simulink model "nn_fuel_control_4_20"  (R2021a)
settings: Solver=ode15s  StartTime=0.0  StopTime=T  MaxStep=.01  RelTol=1e-3
undefined symbols (not defined in the file): AF_sensor_tol, fault_time, fuel_inj_tol, kappa_tol, MAF_sensor_tol, pump_tol, tau_ww_tol
libraries: neural x86
(part 2 of 4)

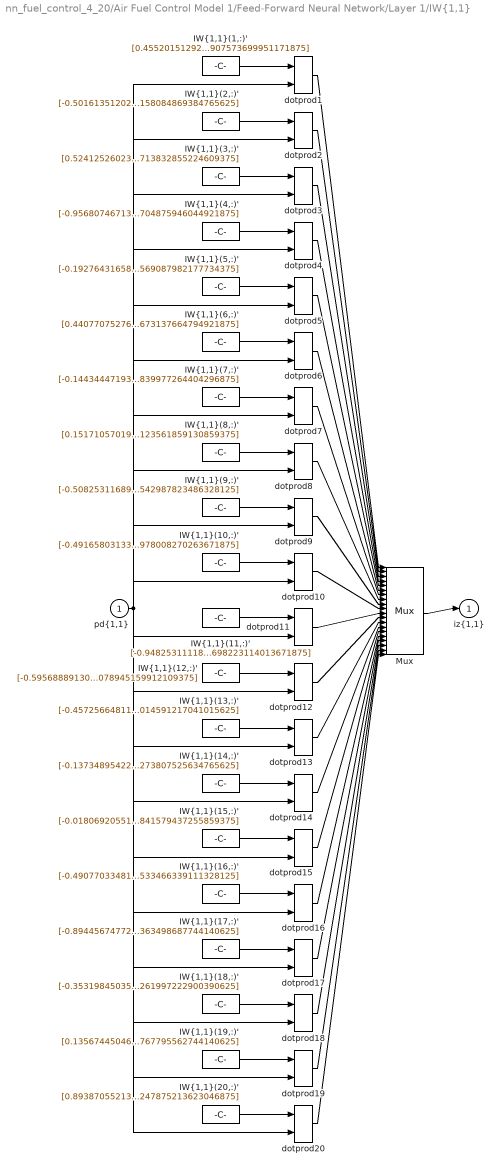
== system nn_fuel_control_4_20/Air Fuel Control Model 1/Feed-Forward Neural Network/Layer 1/IW{1,1} ==
  "pd{1,1}" : Inport  PortDimensions=4
      mask Display: e = 0.06;c1 = [120 230 180]/255;c2 = ([120 230 180]+0)/(256+128);c3 = ([120 230 180]+128)/(256+128);patch([0 1 1 0],[0 0 1 1],c1);patch([0 1 1 1-e 1-e 0+e],[0 0 1 1-e 0+e 0+e],c2);patch([0 0 1 1-e 0+e 0+e],[0 1 1 1-e 1-e 0+e],c3);plot([0 1 1 0 0],[0 0 1 1 0]);
  "IW{1,1}(1,:)'" : Constant  Value=[0.455201512923426532264414845485589466989040374755859375;0.6210675018319438134284382613259367644786834716796875;0.08959089907253227347272428460200899280607700347900390625;1.050437900131484081356347815017215907573699951171875]
      mask Display: e = 0.06;c1 = [120 150 230]/255;c2 = ([120 150 230]+0)/383;c3 = ([120 150 230]+128)/383;patch([0 1 1 0],[0 0 1 1],c1);patch([0 1 1 1-e 1-e 0+e],[0 0 1 1-e 0+e 0+e],c2);patch([0 0 1 1-e 0+e 0+e],[0 1 1 1-e 1-e 0+e],c3);plot([0 1 1 0 0],[0 0 1 1 0]);disp('Weights');
  "IW{1,1}(10,:)'" : Constant  Value=[-0.4916580313329574902780905176769010722637176513671875;0.71234771766081284027904985123313963413238525390625;-0.7859957167075719564053315480123274028301239013671875;0.114661304117702922411581312189809978008270263671875]
      mask Display: e = 0.06;c1 = [120 150 230]/255;c2 = ([120 150 230]+0)/383;c3 = ([120 150 230]+128)/383;patch([0 1 1 0],[0 0 1 1],c1);patch([0 1 1 1-e 1-e 0+e],[0 0 1 1-e 0+e 0+e],c2);patch([0 0 1 1-e 0+e 0+e],[0 1 1 1-e 1-e 0+e],c3);plot([0 1 1 0 0],[0 0 1 1 0]);disp('Weights');
  "IW{1,1}(11,:)'" : Constant  Value=[-0.9482531111801184575682555077946744859218597412109375;0.48788166885906480985113375936634838581085205078125;-0.87517942770330936497202856116928160190582275390625;0.5022120925968749372003685493837110698223114013671875]
      mask Display: e = 0.06;c1 = [120 150 230]/255;c2 = ([120 150 230]+0)/383;c3 = ([120 150 230]+128)/383;patch([0 1 1 0],[0 0 1 1],c1);patch([0 1 1 1-e 1-e 0+e],[0 0 1 1-e 0+e 0+e],c2);patch([0 0 1 1-e 0+e 0+e],[0 1 1 1-e 1-e 0+e],c3);plot([0 1 1 0 0],[0 0 1 1 0]);disp('Weights');
  "IW{1,1}(12,:)'" : Constant  Value=[-0.59568889130134561327167830313555896282196044921875;0.3387998983611222314493716112338006496429443359375;0.009359495090498715086368974880315363407135009765625;-0.4969588631373615950082012204802595078945159912109375]
      mask Display: e = 0.06;c1 = [120 150 230]/255;c2 = ([120 150 230]+0)/383;c3 = ([120 150 230]+128)/383;patch([0 1 1 0],[0 0 1 1],c1);patch([0 1 1 1-e 1-e 0+e],[0 0 1 1-e 0+e 0+e],c2);patch([0 0 1 1-e 0+e 0+e],[0 1 1 1-e 1-e 0+e],c3);plot([0 1 1 0 0],[0 0 1 1 0]);disp('Weights');
  "IW{1,1}(13,:)'" : Constant  Value=[-0.457256648119046371636642334124189801514148712158203125;0.357249947753426611019023084736545570194721221923828125;-0.57752587680887235155324788138386793434619903564453125;0.8892340081964162923355843304307200014591217041015625]
      mask Display: e = 0.06;c1 = [120 150 230]/255;c2 = ([120 150 230]+0)/383;c3 = ([120 150 230]+128)/383;patch([0 1 1 0],[0 0 1 1],c1);patch([0 1 1 1-e 1-e 0+e],[0 0 1 1-e 0+e 0+e],c2);patch([0 0 1 1-e 0+e 0+e],[0 1 1 1-e 1-e 0+e],c3);plot([0 1 1 0 0],[0 0 1 1 0]);disp('Weights');
  "IW{1,1}(14,:)'" : Constant  Value=[-0.1373489542293671039629998631426133215427398681640625;-0.5775747421829160455075680147274397313594818115234375;-0.738357415907519243347678639111109077930450439453125;-0.697311127666600416574738119379617273807525634765625]
      mask Display: e = 0.06;c1 = [120 150 230]/255;c2 = ([120 150 230]+0)/383;c3 = ([120 150 230]+128)/383;patch([0 1 1 0],[0 0 1 1],c1);patch([0 1 1 1-e 1-e 0+e],[0 0 1 1-e 0+e 0+e],c2);patch([0 0 1 1-e 0+e 0+e],[0 1 1 1-e 1-e 0+e],c3);plot([0 1 1 0 0],[0 0 1 1 0]);disp('Weights');
  "IW{1,1}(15,:)'" : Constant  Value=[-0.0180692055168433750311773877683663158677518367767333984375;0.21992142303115691515102980702067725360393524169921875;0.1282003875108993773412890959662036038935184478759765625;0.259471893671093523092707755495212040841579437255859375]
      mask Display: e = 0.06;c1 = [120 150 230]/255;c2 = ([120 150 230]+0)/383;c3 = ([120 150 230]+128)/383;patch([0 1 1 0],[0 0 1 1],c1);patch([0 1 1 1-e 1-e 0+e],[0 0 1 1-e 0+e 0+e],c2);patch([0 0 1 1-e 0+e 0+e],[0 1 1 1-e 1-e 0+e],c3);plot([0 1 1 0 0],[0 0 1 1 0]);disp('Weights');
  "IW{1,1}(16,:)'" : Constant  Value=[-0.4907703348185261660319156362675130367279052734375;-0.0863636826544158520135852086241357028484344482421875;-0.960556512884881197322783918934874236583709716796875;-0.0353694437489793234163926172186620533466339111328125]
      mask Display: e = 0.06;c1 = [120 150 230]/255;c2 = ([120 150 230]+0)/383;c3 = ([120 150 230]+128)/383;patch([0 1 1 0],[0 0 1 1],c1);patch([0 1 1 1-e 1-e 0+e],[0 0 1 1-e 0+e 0+e],c2);patch([0 0 1 1-e 0+e 0+e],[0 1 1 1-e 1-e 0+e],c3);plot([0 1 1 0 0],[0 0 1 1 0]);disp('Weights');
  "IW{1,1}(17,:)'" : Constant  Value=[-0.8944567477260270127459307332173921167850494384765625;-0.74001304047881399927888423917465843260288238525390625;-0.158439343135515942062596650430350564420223236083984375;0.5537273793157526657893185983994044363498687744140625]
      mask Display: e = 0.06;c1 = [120 150 230]/255;c2 = ([120 150 230]+0)/383;c3 = ([120 150 230]+128)/383;patch([0 1 1 0],[0 0 1 1],c1);patch([0 1 1 1-e 1-e 0+e],[0 0 1 1-e 0+e 0+e],c2);patch([0 0 1 1-e 0+e 0+e],[0 1 1 1-e 1-e 0+e],c3);plot([0 1 1 0 0],[0 0 1 1 0]);disp('Weights');
  "IW{1,1}(18,:)'" : Constant  Value=[-0.353198450357381066311290851444937288761138916015625;0.325674444826059339419543903204612433910369873046875;-0.9634401645374384148823310169973410665988922119140625;-0.0229134503222321317394971629255451261997222900390625]
      mask Display: e = 0.06;c1 = [120 150 230]/255;c2 = ([120 150 230]+0)/383;c3 = ([120 150 230]+128)/383;patch([0 1 1 0],[0 0 1 1],c1);patch([0 1 1 1-e 1-e 0+e],[0 0 1 1-e 0+e 0+e],c2);patch([0 0 1 1-e 0+e 0+e],[0 1 1 1-e 1-e 0+e],c3);plot([0 1 1 0 0],[0 0 1 1 0]);disp('Weights');
  "IW{1,1}(19,:)'" : Constant  Value=[0.135674450466279516991363607303355820477008819580078125;-0.549322912787994166450289412750862538814544677734375;-0.471953594740415038888414756002021022140979766845703125;0.1558695073946478049098374185632565058767795562744140625]
      mask Display: e = 0.06;c1 = [120 150 230]/255;c2 = ([120 150 230]+0)/383;c3 = ([120 150 230]+128)/383;patch([0 1 1 0],[0 0 1 1],c1);patch([0 1 1 1-e 1-e 0+e],[0 0 1 1-e 0+e 0+e],c2);patch([0 0 1 1-e 0+e 0+e],[0 1 1 1-e 1-e 0+e],c3);plot([0 1 1 0 0],[0 0 1 1 0]);disp('Weights');
  "IW{1,1}(2,:)'" : Constant  Value=[-0.50161351202444370844801824205205775797367095947265625;0.958190578215499133563071154640056192874908447265625;-0.056301596982187458728663642659739707596600055694580078125;0.040480469393256370003175703686792985536158084869384765625]
      mask Display: e = 0.06;c1 = [120 150 230]/255;c2 = ([120 150 230]+0)/383;c3 = ([120 150 230]+128)/383;patch([0 1 1 0],[0 0 1 1],c1);patch([0 1 1 1-e 1-e 0+e],[0 0 1 1-e 0+e 0+e],c2);patch([0 0 1 1-e 0+e 0+e],[0 1 1 1-e 1-e 0+e],c3);plot([0 1 1 0 0],[0 0 1 1 0]);disp('Weights');
  "IW{1,1}(20,:)'" : Constant  Value=[0.8938705521315066793164305636310018599033355712890625;0.96329793238814798161939734200132079422473907470703125;-0.295572392642879544499834310045116581022739410400390625;0.87909372842644284418156530591659247875213623046875]
      mask Display: e = 0.06;c1 = [120 150 230]/255;c2 = ([120 150 230]+0)/383;c3 = ([120 150 230]+128)/383;patch([0 1 1 0],[0 0 1 1],c1);patch([0 1 1 1-e 1-e 0+e],[0 0 1 1-e 0+e 0+e],c2);patch([0 0 1 1-e 0+e 0+e],[0 1 1 1-e 1-e 0+e],c3);plot([0 1 1 0 0],[0 0 1 1 0]);disp('Weights');
  "IW{1,1}(3,:)'" : Constant  Value=[0.5241252602301378349380911458865739405155181884765625;0.8167734373000536951536787455552257597446441650390625;-0.74201764338017017763604599167592823505401611328125;-0.832946956754459844063376294798217713832855224609375]
      mask Display: e = 0.06;c1 = [120 150 230]/255;c2 = ([120 150 230]+0)/383;c3 = ([120 150 230]+128)/383;patch([0 1 1 0],[0 0 1 1],c1);patch([0 1 1 1-e 1-e 0+e],[0 0 1 1-e 0+e 0+e],c2);patch([0 0 1 1-e 0+e 0+e],[0 1 1 1-e 1-e 0+e],c3);plot([0 1 1 0 0],[0 0 1 1 0]);disp('Weights');
  "IW{1,1}(4,:)'" : Constant  Value=[-0.956807467135799782909089117310941219329833984375;-0.0493903087290285258692534853253164328634738922119140625;-0.9415456718123842438927795228664763271808624267578125;-0.030347378954881314150338056379041518084704875946044921875]
      mask Display: e = 0.06;c1 = [120 150 230]/255;c2 = ([120 150 230]+0)/383;c3 = ([120 150 230]+128)/383;patch([0 1 1 0],[0 0 1 1],c1);patch([0 1 1 1-e 1-e 0+e],[0 0 1 1-e 0+e 0+e],c2);patch([0 0 1 1-e 0+e 0+e],[0 1 1 1-e 1-e 0+e],c3);plot([0 1 1 0 0],[0 0 1 1 0]);disp('Weights');
  "IW{1,1}(5,:)'" : Constant  Value=[-0.192764316586044592849447099069948308169841766357421875;-0.68996992127067391376016303183860145509243011474609375;0.354029156232344377475129704180289991199970245361328125;-0.08997556570563967903719770902171148918569087982177734375]
      mask Display: e = 0.06;c1 = [120 150 230]/255;c2 = ([120 150 230]+0)/383;c3 = ([120 150 230]+128)/383;patch([0 1 1 0],[0 0 1 1],c1);patch([0 1 1 1-e 1-e 0+e],[0 0 1 1-e 0+e 0+e],c2);patch([0 0 1 1-e 0+e 0+e],[0 1 1 1-e 1-e 0+e],c3);plot([0 1 1 0 0],[0 0 1 1 0]);disp('Weights');
  "IW{1,1}(6,:)'" : Constant  Value=[0.440770752766682705203749037536908872425556182861328125;0.1872641645973948387737806342556723393499851226806640625;0.46877269832112744563090700467000715434551239013671875;0.09773402402077450978890027499801362864673137664794921875]
      mask Display: e = 0.06;c1 = [120 150 230]/255;c2 = ([120 150 230]+0)/383;c3 = ([120 150 230]+128)/383;patch([0 1 1 0],[0 0 1 1],c1);patch([0 1 1 1-e 1-e 0+e],[0 0 1 1-e 0+e 0+e],c2);patch([0 0 1 1-e 0+e 0+e],[0 1 1 1-e 1-e 0+e],c3);plot([0 1 1 0 0],[0 0 1 1 0]);disp('Weights');
  "IW{1,1}(7,:)'" : Constant  Value=[-0.1443444719366482609235191603147541172802448272705078125;0.142050703362333441415188417522585950791835784912109375;-0.81241480909466534665597237108158878982067108154296875;-0.37841350313330568422287569774198345839977264404296875]
      mask Display: e = 0.06;c1 = [120 150 230]/255;c2 = ([120 150 230]+0)/383;c3 = ([120 150 230]+128)/383;patch([0 1 1 0],[0 0 1 1],c1);patch([0 1 1 1-e 1-e 0+e],[0 0 1 1-e 0+e 0+e],c2);patch([0 0 1 1-e 0+e 0+e],[0 1 1 1-e 1-e 0+e],c3);plot([0 1 1 0 0],[0 0 1 1 0]);disp('Weights');
  "IW{1,1}(8,:)'" : Constant  Value=[0.1517105701921201699189367673170636408030986785888671875;0.1730723960461933164101111515265074558556079864501953125;-0.51555047379194707257710206249612383544445037841796875;0.54893240153364286637582836192450486123561859130859375]
      mask Display: e = 0.06;c1 = [120 150 230]/255;c2 = ([120 150 230]+0)/383;c3 = ([120 150 230]+128)/383;patch([0 1 1 0],[0 0 1 1],c1);patch([0 1 1 1-e 1-e 0+e],[0 0 1 1-e 0+e 0+e],c2);patch([0 0 1 1-e 0+e 0+e],[0 1 1 1-e 1-e 0+e],c3);plot([0 1 1 0 0],[0 0 1 1 0]);disp('Weights');
  "IW{1,1}(9,:)'" : Constant  Value=[-0.5082531168947779232070161015144549310207366943359375;-0.2024999076040734369286155924783088266849517822265625;0.40301013753805303707622442743740975856781005859375;-0.1068582787601883854478046487201936542987823486328125]
      mask Display: e = 0.06;c1 = [120 150 230]/255;c2 = ([120 150 230]+0)/383;c3 = ([120 150 230]+128)/383;patch([0 1 1 0],[0 0 1 1],c1);patch([0 1 1 1-e 1-e 0+e],[0 0 1 1-e 0+e 0+e],c2);patch([0 0 1 1-e 0+e 0+e],[0 1 1 1-e 1-e 0+e],c3);plot([0 1 1 0 0],[0 0 1 1 0]);disp('Weights');
  Mux : Mux  Inputs=20
      mask Display: e = 0.06;c1 = [120 150 230]/255;c2 = ([120 150 230]+0)/383;c3 = ([120 150 230]+128)/383;patch([0 1 1 0],[0 0 1 1],c1);patch([0 1 1 1-e 1-e 0+e],[0 0 1 1-e 0+e 0+e],c2);patch([0 0 1 1-e 0+e 0+e],[0 1 1 1-e 1-e 0+e],c3);plot([0 1 1 0 0],[0 0 1 1 0]);disp('Mux');
  dotprod{1..20} (20 alike) : neural/Weight Functions/dotprod
  "iz{1,1}" : Outport
      mask Display: e = 0.06;c1 = [120 230 180]/255;c2 = ([120 230 180]+0)/(256+128);c3 = ([120 230 180]+128)/(256+128);patch([0 1 1 0],[0 0 1 1],c1);patch([0 1 1 1-e 1-e 0+e],[0 0 1 1-e 0+e 0+e],c2);patch([0 0 1 1-e 0+e 0+e],[0 1 1 1-e 1-e 0+e],c3);plot([0 1 1 0 0],[0 0 1 1 0]);
  wires:
  "IW{1,1}(1,:)'"/1 -> dotprod1/1
  "pd{1,1}"/1 -> dotprod1/2, dotprod2/2, dotprod3/2, dotprod4/2, dotprod5/2, dotprod6/2, dotprod7/2, dotprod8/2, dotprod9/2, dotprod10/2, dotprod11/2, dotprod12/2, dotprod13/2, dotprod14/2, dotprod15/2, dotprod16/2, dotprod17/2, dotprod18/2, dotprod19/2, dotprod20/2
  dotprod1/1 -> Mux/1
  "IW{1,1}(2,:)'"/1 -> dotprod2/1
  dotprod2/1 -> Mux/2
  "IW{1,1}(3,:)'"/1 -> dotprod3/1
  dotprod3/1 -> Mux/3
  "IW{1,1}(4,:)'"/1 -> dotprod4/1
  dotprod4/1 -> Mux/4
  "IW{1,1}(5,:)'"/1 -> dotprod5/1
  dotprod5/1 -> Mux/5
  "IW{1,1}(6,:)'"/1 -> dotprod6/1
  dotprod6/1 -> Mux/6
  "IW{1,1}(7,:)'"/1 -> dotprod7/1
  dotprod7/1 -> Mux/7
  "IW{1,1}(8,:)'"/1 -> dotprod8/1
  dotprod8/1 -> Mux/8
  "IW{1,1}(9,:)'"/1 -> dotprod9/1
  dotprod9/1 -> Mux/9
  "IW{1,1}(10,:)'"/1 -> dotprod10/1
  dotprod10/1 -> Mux/10
  "IW{1,1}(11,:)'"/1 -> dotprod11/1
  dotprod11/1 -> Mux/11
  "IW{1,1}(12,:)'"/1 -> dotprod12/1
  dotprod12/1 -> Mux/12
  "IW{1,1}(13,:)'"/1 -> dotprod13/1
  dotprod13/1 -> Mux/13
  "IW{1,1}(14,:)'"/1 -> dotprod14/1
  dotprod14/1 -> Mux/14
  "IW{1,1}(15,:)'"/1 -> dotprod15/1
  dotprod15/1 -> Mux/15
  "IW{1,1}(16,:)'"/1 -> dotprod16/1
  dotprod16/1 -> Mux/16
  "IW{1,1}(17,:)'"/1 -> dotprod17/1
  dotprod17/1 -> Mux/17
  "IW{1,1}(18,:)'"/1 -> dotprod18/1
  dotprod18/1 -> Mux/18
  "IW{1,1}(19,:)'"/1 -> dotprod19/1
  dotprod19/1 -> Mux/19
  "IW{1,1}(20,:)'"/1 -> dotprod20/1
  dotprod20/1 -> Mux/20
  Mux/1 -> "iz{1,1}"/1

== system nn_fuel_control_4_20/Air Fuel Control Model 1/Feed-Forward Neural Network/Layer 2/Delays 1 ==
  "p{2}" : Inport  PortDimensions=20
      mask Display: e = 0.06;c1 = [120 230 180]/255;c2 = ([120 230 180]+0)/(256+128);c3 = ([120 230 180]+128)/(256+128);patch([0 1 1 0],[0 0 1 1],c1);patch([0 1 1 1-e 1-e 0+e],[0 0 1 1-e 0+e 0+e],c2);patch([0 0 1 1-e 0+e 0+e],[0 1 1 1-e 1-e 0+e],c3);plot([0 1 1 0 0],[0 0 1 1 0]);
  mux : Mux  Inputs=1
      mask Display: e = 0.06;c1 = [120 150 230]/255;c2 = ([120 150 230]+0)/383;c3 = ([120 150 230]+128)/383;patch([0 1 1 0],[0 0 1 1],c1);patch([0 1 1 1-e 1-e 0+e],[0 0 1 1-e 0+e 0+e],c2);patch([0 0 1 1-e 0+e 0+e],[0 1 1 1-e 1-e 0+e],c3);plot([0 1 1 0 0],[0 0 1 1 0]);disp('Mux')
  "pd{2,1}" : Outport
      mask Display: e = 0.06;c1 = [120 230 180]/255;c2 = ([120 230 180]+0)/(256+128);c3 = ([120 230 180]+128)/(256+128);patch([0 1 1 0],[0 0 1 1],c1);patch([0 1 1 1-e 1-e 0+e],[0 0 1 1-e 0+e 0+e],c2);patch([0 0 1 1-e 0+e 0+e],[0 1 1 1-e 1-e 0+e],c3);plot([0 1 1 0 0],[0 0 1 1 0]);
  wires:
  "p{2}"/1 -> mux/1
  mux/1 -> "pd{2,1}"/1

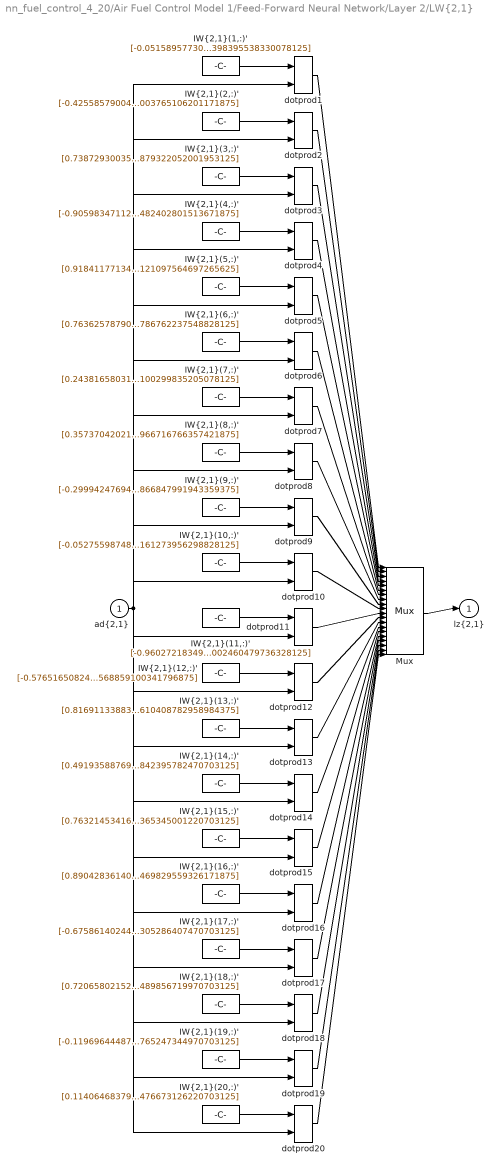
== system nn_fuel_control_4_20/Air Fuel Control Model 1/Feed-Forward Neural Network/Layer 2/LW{2,1} ==
  "ad{2,1}" : Inport  PortDimensions=20
      mask Display: e = 0.06;c1 = [120 230 180]/255;c2 = ([120 230 180]+0)/(256+128);c3 = ([120 230 180]+128)/(256+128);patch([0 1 1 0],[0 0 1 1],c1);patch([0 1 1 1-e 1-e 0+e],[0 0 1 1-e 0+e 0+e],c2);patch([0 0 1 1-e 0+e 0+e],[0 1 1 1-e 1-e 0+e],c3);plot([0 1 1 0 0],[0 0 1 1 0]);
  "IW{2,1}(1,:)'" : Constant  Value=[-0.05158957730929480955950339193805120885372161865234375;0.005653175358640328239390182574197751819156110286712646484375;0.823713516811877877188408092479221522808074951171875;0.26105981244798837082043974078260362148284912109375;0.3363752213625745834946201284765265882015228271484375;0.007301814495751283995428337902922066859900951385498046875;0.942430881921875407414290748420171439647674560546875;0.2302164082627291830096538660654914565384387969970703125;0.7225781228481757967330167957697995007038116455078125;-0.55903537873570652294574756524525582790374755859375;0.3468810802850585961465412765392102301120758056640625;0.4787282035194555529500348711735568940639495849609375;0.105449017197976668835934788148733787238597869873046875;0.305593703721999787603635923005640506744384765625;-0.402804836675209887442150602510082535445690155029296875;-0.38658905442980451283574439003132283687591552734375;0.040096726165785197271151929498955723829567432403564453125;-0.357109696841054091720479846117086708545684814453125;0.0668979846995910454321432325741625390946865081787109375;0.9293358122750270400302952111815102398395538330078125]
      mask Display: e = 0.06;c1 = [120 150 230]/255;c2 = ([120 150 230]+0)/383;c3 = ([120 150 230]+128)/383;patch([0 1 1 0],[0 0 1 1],c1);patch([0 1 1 1-e 1-e 0+e],[0 0 1 1-e 0+e 0+e],c2);patch([0 0 1 1-e 0+e 0+e],[0 1 1 1-e 1-e 0+e],c3);plot([0 1 1 0 0],[0 0 1 1 0]);disp('weights');
  "IW{2,1}(10,:)'" : Constant  Value=[-0.05275598748487618505631502330288640223443508148193359375;0.308898904971982524170215356207336299121379852294921875;-0.653212901425074488059863142552785575389862060546875;-0.8129162492509938164886307276901789009571075439453125;0.78123078673014401118734895135276019573211669921875;-0.866190723055696221166499526589177548885345458984375;0.738309357231496488083166696014814078807830810546875;0.61676355332865850922274830736569128930568695068359375;0.1629757095855435267139910138212144374847412109375;-0.088014573433287335291197450715117156505584716796875;0.1263945153746492966462255935766734182834625244140625;-0.7242413034889867429200194237637333571910858154296875;-0.6992811158873866173024680392700247466564178466796875;-0.882059250596157529145102671463973820209503173828125;-0.57218102927048131167708788780146278440952301025390625;-0.18259363205784584494040245772339403629302978515625;0.022114677854097652964782128037768416106700897216796875;-0.8559234116054577068410935680731199681758880615234375;0.7490243659842532597537001493037678301334381103515625;-0.393452895879057351624652483224053867161273956298828125]
      mask Display: e = 0.06;c1 = [120 150 230]/255;c2 = ([120 150 230]+0)/383;c3 = ([120 150 230]+128)/383;patch([0 1 1 0],[0 0 1 1],c1);patch([0 1 1 1-e 1-e 0+e],[0 0 1 1-e 0+e 0+e],c2);patch([0 0 1 1-e 0+e 0+e],[0 1 1 1-e 1-e 0+e],c3);plot([0 1 1 0 0],[0 0 1 1 0]);disp('weights');
  "IW{2,1}(11,:)'" : Constant  Value=[-0.9602721834970935343989140164921991527080535888671875;0.70877657591812270876374668659991584718227386474609375;0.5741210688958588992392151340027339756488800048828125;0.08830282490748629642407507844836800359189510345458984375;0.9169479943996492465885239653289318084716796875;-0.77586282164734854394083640727330930531024932861328125;0.10227348148213437351028431976374122314155101776123046875;0.73766298661537776926166998237022198736667633056640625;0.2678569611350223311774243484251201152801513671875;0.8608424021435674422519923609797842800617218017578125;0.3856132299752932368619440239854156970977783203125;-0.5802490370587134460578226935467682778835296630859375;0.470376658928852109387008795238216407597064971923828125;0.4438431689988495687515523968613706529140472412109375;0.84843293500289196362729171596583910286426544189453125;-0.44530489605756873316977362264879047870635986328125;-0.279710890733623707138377767478232271969318389892578125;-0.9971046456737548968618511935346759855747222900390625;0.1689951293922603847708074908950948156416416168212890625;0.430252247013837518796464109982480295002460479736328125]
      mask Display: e = 0.06;c1 = [120 150 230]/255;c2 = ([120 150 230]+0)/383;c3 = ([120 150 230]+128)/383;patch([0 1 1 0],[0 0 1 1],c1);patch([0 1 1 1-e 1-e 0+e],[0 0 1 1-e 0+e 0+e],c2);patch([0 0 1 1-e 0+e 0+e],[0 1 1 1-e 1-e 0+e],c3);plot([0 1 1 0 0],[0 0 1 1 0]);disp('weights');
  "IW{2,1}(12,:)'" : Constant  Value=[-0.57651650824180389331985452372464351356029510498046875;0.250358835331461027084998249847558327019214630126953125;-0.219198035136920932330895084305666387081146240234375;-0.09375054463766839540905806416049017570912837982177734375;0.5252040261281705202378589092404581606388092041015625;-0.000319211106394178532365268896597854109131731092929840087890625;-0.473674377494609777361489477698341943323612213134765625;0.6018290141493987110976604526513256132602691650390625;-0.2868412803874023087047362423618324100971221923828125;-0.9428484444955078647154778082040138542652130126953125;-0.46388239418073595743408077396452426910400390625;-0.65804280535339554347729063010774552822113037109375;-0.058815418926318606407388500656452379189431667327880859375;-0.0057849695429974534732764368527568876743316650390625;0.2961529404426730405219814201700501143932342529296875;0.3970770210515313092258793403743766248226165771484375;0.693432755278055257264213651069439947605133056640625;-0.1708604503139026231650632325909100472927093505859375;0.392601119147283517119007001383579336106777191162109375;-0.40474212818124033486100188383716158568859100341796875]
      mask Display: e = 0.06;c1 = [120 150 230]/255;c2 = ([120 150 230]+0)/383;c3 = ([120 150 230]+128)/383;patch([0 1 1 0],[0 0 1 1],c1);patch([0 1 1 1-e 1-e 0+e],[0 0 1 1-e 0+e 0+e],c2);patch([0 0 1 1-e 0+e 0+e],[0 1 1 1-e 1-e 0+e],c3);plot([0 1 1 0 0],[0 0 1 1 0]);disp('weights');
  "IW{2,1}(13,:)'" : Constant  Value=[0.816911338830066835470233854721300303936004638671875;-0.27269698140621512205683529828093014657497406005859375;0.477633731697185037745612135040573775768280029296875;-0.11982998674005938821718331155352643691003322601318359375;-0.468577371179003054901812674870598129928112030029296875;-0.83042310620928727615819298080168664455413818359375;-0.2346229414290626202888034868010436184704303741455078125;-0.1320780419089263302279135814387700520455837249755859375;0.8883496982022638377429757383652031421661376953125;-0.8880833329269346432255360923591069877147674560546875;-0.7351930155494545982008958162623457610607147216796875;0.65209150290458151033590183942578732967376708984375;0.70910927909142740244163860552362166345119476318359375;-0.080367458233499888820006162859499454498291015625;0.7463764861435671083000897851889021694660186767578125;-0.5159764351431530560176952349138446152210235595703125;0.91422033592877649521568628188106231391429901123046875;-0.9364660874875536666905873062205500900745391845703125;0.91827566768034241118101590473088435828685760498046875;-0.1656505772563306722044984553576796315610408782958984375]
      mask Display: e = 0.06;c1 = [120 150 230]/255;c2 = ([120 150 230]+0)/383;c3 = ([120 150 230]+128)/383;patch([0 1 1 0],[0 0 1 1],c1);patch([0 1 1 1-e 1-e 0+e],[0 0 1 1-e 0+e 0+e],c2);patch([0 0 1 1-e 0+e 0+e],[0 1 1 1-e 1-e 0+e],c3);plot([0 1 1 0 0],[0 0 1 1 0]);disp('weights');
  "IW{2,1}(14,:)'" : Constant  Value=[0.49193588769640916869008151479647494852542877197265625;-0.41808437171363710405103120137937366962432861328125;0.0381627451031614217669130084686912596225738525390625;0.75151351881049344161311864809249527752399444580078125;-0.95710459906888456504958639925462193787097930908203125;0.131027644957525613023108235211111605167388916015625;-0.348824693553620779340462831896729767322540283203125;0.6754591907370313119685079072951339185237884521484375;-0.75679949900757836900311303907074034214019775390625;0.3720487521166280231454948079772293567657470703125;-0.1936175322065689652362152628484182059764862060546875;0.779304712714375735771454856148920953273773193359375;0.493635496942827323163527353244717232882976531982421875;-0.0970747772544691134299910117988474667072296142578125;-0.475718106478187741092966689393506385385990142822265625;0.442287295486071041494824385154061019420623779296875;-0.10022331843492175706966662573904613964259624481201171875;-0.875045011654159043956724417512305080890655517578125;0.361402217707740558427786936590564437210559844970703125;0.6061119968902428656321035305154509842395782470703125]
      mask Display: e = 0.06;c1 = [120 150 230]/255;c2 = ([120 150 230]+0)/383;c3 = ([120 150 230]+128)/383;patch([0 1 1 0],[0 0 1 1],c1);patch([0 1 1 1-e 1-e 0+e],[0 0 1 1-e 0+e 0+e],c2);patch([0 0 1 1-e 0+e 0+e],[0 1 1 1-e 1-e 0+e],c3);plot([0 1 1 0 0],[0 0 1 1 0]);disp('weights');
  "IW{2,1}(15,:)'" : Constant  Value=[0.7632145341614713363043165372801013290882110595703125;-0.54035110201968705734287823361228220164775848388671875;0.99496333243500334475584168103523552417755126953125;-0.41643452764151589473584635925362817943096160888671875;-0.81176838714621257775405638312804512679576873779296875;0.378555997344059369513757928871200419962406158447265625;-0.7562928430067541452075374763808213174343109130859375;0.22897082021425674280834527962724678218364715576171875;-0.424662035581437447007147056865505874156951904296875;0.5488774207235953550565454861498437821865081787109375;-0.613178793930092336239567885058932006359100341796875;0.31332364621904051915635136538185179233551025390625;0.279556466629975963744669797961250878870487213134765625;0.7570679251397149922553353462717495858669281005859375;0.96659387647248384833886802880442701280117034912109375;-0.1431939639002364206277206903905607759952545166015625;0.1266749077172355242293377841633628122508525848388671875;-0.030277693910024883194864742108620703220367431640625;0.31753139396024609997226662017055787146091461181640625;0.304140586887838904051051258647930808365345001220703125]
      mask Display: e = 0.06;c1 = [120 150 230]/255;c2 = ([120 150 230]+0)/383;c3 = ([120 150 230]+128)/383;patch([0 1 1 0],[0 0 1 1],c1);patch([0 1 1 1-e 1-e 0+e],[0 0 1 1-e 0+e 0+e],c2);patch([0 0 1 1-e 0+e 0+e],[0 1 1 1-e 1-e 0+e],c3);plot([0 1 1 0 0],[0 0 1 1 0]);disp('weights');
  "IW{2,1}(16,:)'" : Constant  Value=[0.89042836140007608491941937245428562164306640625;-0.39718317008346193386358891075360588729381561279296875;0.7216422349541506964243353650090284645557403564453125;-0.68059865039962075261570362272323109209537506103515625;0.424569985203905708726068723990465514361858367919921875;0.79291073974151327075077233530464582145214080810546875;0.0858037118521310093743892366546788252890110015869140625;0.329336111039964907210020328420796431601047515869140625;0.3972561322452710097508088438189588487148284912109375;0.556694552801444419998233570368029177188873291015625;0.939275970334976673115079393028281629085540771484375;0.5407559792593226166701469992403872311115264892578125;-0.66086530482279048914762142885592766106128692626953125;-0.8856326487327705887508955129305832087993621826171875;0.77924910822132054111222032588557340204715728759765625;-0.4560217201167635625580487612751312553882598876953125;0.59835034564828626368893083053990267217159271240234375;0.4800795410237679305964775267057120800018310546875;-0.7604867205853482747812677189358510076999664306640625;-0.14593469566804528891879044749657623469829559326171875]
      mask Display: e = 0.06;c1 = [120 150 230]/255;c2 = ([120 150 230]+0)/383;c3 = ([120 150 230]+128)/383;patch([0 1 1 0],[0 0 1 1],c1);patch([0 1 1 1-e 1-e 0+e],[0 0 1 1-e 0+e 0+e],c2);patch([0 0 1 1-e 0+e 0+e],[0 1 1 1-e 1-e 0+e],c3);plot([0 1 1 0 0],[0 0 1 1 0]);disp('weights');
  "IW{2,1}(17,:)'" : Constant  Value=[-0.6758614024478462045664173274417407810688018798828125;-0.5358077941627923390655041657737456262111663818359375;-0.9302654717113429949648661931860260665416717529296875;0.0584786707709918918141056565218605101108551025390625;-0.1563535073477628767335545489913783967494964599609375;-0.1698033685133155668012250316678546369075775146484375;0.641294048833410013088496270938776433467864990234375;-0.8482768551888189012544216893729753792285919189453125;-0.73926280341947769869648254825733602046966552734375;-0.60654927412420978072304933448322117328643798828125;-0.3207823148820490022359308568411506712436676025390625;0.7286371347762752304078048837254755198955535888671875;0.221161711610812883321841582073830068111419677734375;-0.3135444716324717884248229893273673951625823974609375;-0.20231351574388600766951640252955257892608642578125;0.02004847836207801492491853423416614532470703125;-0.5205462910234504025908108815201558172702789306640625;-0.3419510647345320730750017901300452649593353271484375;-0.7552936880422418397529327194206416606903076171875;-0.36831387560758077626132944715209305286407470703125]
      mask Display: e = 0.06;c1 = [120 150 230]/255;c2 = ([120 150 230]+0)/383;c3 = ([120 150 230]+128)/383;patch([0 1 1 0],[0 0 1 1],c1);patch([0 1 1 1-e 1-e 0+e],[0 0 1 1-e 0+e 0+e],c2);patch([0 0 1 1-e 0+e 0+e],[0 1 1 1-e 1-e 0+e],c3);plot([0 1 1 0 0],[0 0 1 1 0]);disp('weights');
  "IW{2,1}(18,:)'" : Constant  Value=[0.7206580215290363522484540226287208497524261474609375;0.321782865135176177062703573028557002544403076171875;0.0709256267373914450757865779451094567775726318359375;0.2521402991659267289747958784573711454868316650390625;-0.501748435262526104594371645362116396427154541015625;-0.819907001970385795885931656812317669391632080078125;0.840435083719567099791447617462836205959320068359375;0.1445774483427773038357599943992681801319122314453125;-0.3644268991194905549235727448831312358379364013671875;0.4089785597889472601451643640757538378238677978515625;-0.537795497440453740267685134313069283962249755859375;0.98903102999879610734978996333666145801544189453125;0.4182435879757175900550691949320025742053985595703125;0.3377585324774112773837941858801059424877166748046875;-0.46367148500896337992571716313250362873077392578125;0.4829290609627052699437399496673606336116790771484375;-0.5564821986119075081234086610493250191211700439453125;0.05341436384908160306395075167529284954071044921875;0.84643171578021192402729866444133222103118896484375;-0.606182820890265094959659109008498489856719970703125]
      mask Display: e = 0.06;c1 = [120 150 230]/255;c2 = ([120 150 230]+0)/383;c3 = ([120 150 230]+128)/383;patch([0 1 1 0],[0 0 1 1],c1);patch([0 1 1 1-e 1-e 0+e],[0 0 1 1-e 0+e 0+e],c2);patch([0 0 1 1-e 0+e 0+e],[0 1 1 1-e 1-e 0+e],c3);plot([0 1 1 0 0],[0 0 1 1 0]);disp('weights');
  "IW{2,1}(19,:)'" : Constant  Value=[-0.1196964448752895204819424179731868207454681396484375;-0.6727120731846600865111440725740976631641387939453125;-0.1717583668323487966489437894779257476329803466796875;0.7100819252171446382959629772813059389591217041015625;-0.3555076206573091202045588943292386829853057861328125;0.8647490254675478382750952732749283313751220703125;0.22874332639720051929543842561542987823486328125;0.8264065275737355609209089379874058067798614501953125;-0.8991179105813944527625380942481569945812225341796875;0.5555430023846443798873906416702084243297576904296875;0.5359794795115229160131775643094442784786224365234375;0.046344409840232803077242351719178259372711181640625;-0.3400567986666518383032098427065648138523101806640625;-0.9882058453176938428441644646227359771728515625;-0.4830885572269856265137377704377286136150360107421875;-0.939236556894458285427162991254590451717376708984375;-0.192238262757973732419713996932841837406158447265625;-0.63143851565173125806040843599475920200347900390625;-0.7632417201889918345614205463789403438568115234375;0.33670387503982812660296985995955765247344970703125]
      mask Display: e = 0.06;c1 = [120 150 230]/255;c2 = ([120 150 230]+0)/383;c3 = ([120 150 230]+128)/383;patch([0 1 1 0],[0 0 1 1],c1);patch([0 1 1 1-e 1-e 0+e],[0 0 1 1-e 0+e 0+e],c2);patch([0 0 1 1-e 0+e 0+e],[0 1 1 1-e 1-e 0+e],c3);plot([0 1 1 0 0],[0 0 1 1 0]);disp('weights');
  "IW{2,1}(2,:)'" : Constant  Value=[-0.425585790046403733555280268774367868900299072265625;0.327250814693552438683354921522550284862518310546875;0.7551928234128781891598691800027154386043548583984375;0.8110540085465327564406834426335990428924560546875;-0.4441935652485164975900033823563717305660247802734375;-0.9204076215466319155211749603040516376495361328125;0.8552907975471517598720083697116933763027191162109375;-0.9887734046260743259182390829664655029773712158203125;0.357454319626427707845550685306079685688018798828125;0.4593662043034421049725324337487109005451202392578125;0.9794337819448795112720063116285018622875213623046875;0.641773009900934443550113428500480949878692626953125;-0.0891900940331471492328319072839803993701934814453125;-0.5556751745203432069075688559678383171558380126953125;-0.6392964716803390956556540913879871368408203125;0.799616017271743029226627186289988458156585693359375;-0.0135261086921596440646453629597090184688568115234375;-0.2671946669807028218457389812101610004901885986328125;-0.20528182163962416240110542275942862033843994140625;0.306575665526210183742250592331402003765106201171875]
      mask Display: e = 0.06;c1 = [120 150 230]/255;c2 = ([120 150 230]+0)/383;c3 = ([120 150 230]+128)/383;patch([0 1 1 0],[0 0 1 1],c1);patch([0 1 1 1-e 1-e 0+e],[0 0 1 1-e 0+e 0+e],c2);patch([0 0 1 1-e 0+e 0+e],[0 1 1 1-e 1-e 0+e],c3);plot([0 1 1 0 0],[0 0 1 1 0]);disp('weights');
  "IW{2,1}(20,:)'" : Constant  Value=[0.1140646837937922264405443684154306538403034210205078125;-0.48460308795281592519899049875675700604915618896484375;0.2412854964956980818868714777636341750621795654296875;0.132920918826495426667833044120925478637218475341796875;0.271380005536353607897837036944110877811908721923828125;0.571918826538477365062362878234125673770904541015625;0.206706730991620124537888614213443361222743988037109375;0.216462193839773220371824891117285005748271942138671875;-0.3367533904809600908691891163471154868602752685546875;-0.3513001532269355298154778211028315126895904541015625;0.8820274073654716939785203067003749310970306396484375;0.1351981071309131809954351410851813852787017822265625;-0.288653764661439937722064996705739758908748626708984375;-0.6401911504383439588394821839756332337856292724609375;0.83974755662854982940501713528647087514400482177734375;-0.1064239804228097607818881442653946578502655029296875;0.83028969186877821240244657019502483308315277099609375;-0.519207538673606361356860361411236226558685302734375;-0.53720075244854792462234627237194217741489410400390625;0.47981451665761565283929712677490897476673126220703125]
      mask Display: e = 0.06;c1 = [120 150 230]/255;c2 = ([120 150 230]+0)/383;c3 = ([120 150 230]+128)/383;patch([0 1 1 0],[0 0 1 1],c1);patch([0 1 1 1-e 1-e 0+e],[0 0 1 1-e 0+e 0+e],c2);patch([0 0 1 1-e 0+e 0+e],[0 1 1 1-e 1-e 0+e],c3);plot([0 1 1 0 0],[0 0 1 1 0]);disp('weights');
  "IW{2,1}(3,:)'" : Constant  Value=[0.738729300359305174339397126459516584873199462890625;-0.15950300371264358734180177634698338806629180908203125;0.356982538310723906960220119799487292766571044921875;0.82876467959214206171481009732815437018871307373046875;0.77137590845207981704589883520384319126605987548828125;0.3446637959714593524296333271195180714130401611328125;-0.5931892861562368945982370860292576253414154052734375;0.79488184572168785191337292417301796376705169677734375;-0.3983407617695891023146259612985886633396148681640625;0.996905374217900597244579330435954034328460693359375;-0.3854335085292690532554615856497548520565032958984375;0.6774262232416130569134793404373340308666229248046875;0.78286213256441328223189657364855520427227020263671875;0.8128553037420480631425334649975411593914031982421875;0.270540875581002648875283966845017857849597930908203125;0.7010165126864007500984143916866742074489593505859375;0.8988202248689010076532213133759796619415283203125;-0.6440113930643847073298502436955459415912628173828125;-0.019329710689218772279307501094081089831888675689697265625;0.1779482614745891144725220556210842914879322052001953125]
      mask Display: e = 0.06;c1 = [120 150 230]/255;c2 = ([120 150 230]+0)/383;c3 = ([120 150 230]+128)/383;patch([0 1 1 0],[0 0 1 1],c1);patch([0 1 1 1-e 1-e 0+e],[0 0 1 1-e 0+e 0+e],c2);patch([0 0 1 1-e 0+e 0+e],[0 1 1 1-e 1-e 0+e],c3);plot([0 1 1 0 0],[0 0 1 1 0]);disp('weights');
  "IW{2,1}(4,:)'" : Constant  Value=[-0.9059834711213958780007260429556481540203094482421875;0.66240119589044621495332876293105073273181915283203125;-0.4744001172629286333659592855838127434253692626953125;0.3171400911300332747799757271423004567623138427734375;0.5545185935621954609331396568450145423412322998046875;0.215071315658744099952315309565165080130100250244140625;-0.939781925896429726208225474692881107330322265625;0.405976236471921658743866601071204058825969696044921875;-0.83409532270698338862757736933417618274688720703125;-0.2018899267713203382612618952407501637935638427734375;0.6998971334593264703727300002356059849262237548828125;0.8508504199885214003273858907050453126430511474609375;0.52881147412598206170031289730104617774486541748046875;0.7479459577875948728120647501782514154911041259765625;-0.375057415375808000934654273805790580809116363525390625;0.24844320548986242869204943417571485042572021484375;0.00166395997385810853232135375634470619843341410160064697265625;0.9534683196563360496611494454555213451385498046875;0.1677183993692243912931871818727813661098480224609375;0.016135642131118781150700414173115859739482402801513671875]
      mask Display: e = 0.06;c1 = [120 150 230]/255;c2 = ([120 150 230]+0)/383;c3 = ([120 150 230]+128)/383;patch([0 1 1 0],[0 0 1 1],c1);patch([0 1 1 1-e 1-e 0+e],[0 0 1 1-e 0+e 0+e],c2);patch([0 0 1 1-e 0+e 0+e],[0 1 1 1-e 1-e 0+e],c3);plot([0 1 1 0 0],[0 0 1 1 0]);disp('weights');
  "IW{2,1}(5,:)'" : Constant  Value=[0.918411771349174177458962731179781258106231689453125;0.02861710912490078584369257441721856594085693359375;-0.3658001153270580285692403776920400559902191162109375;0.3291407845097251705368535112938843667507171630859375;0.0390353186877276936428415865520946681499481201171875;-0.8950672732069338000115976683446206152439117431640625;-0.0773508899561903273678353798459284007549285888671875;0.4890666829231455903226333248312585055828094482421875;0.6891738745702473689647149512893520295619964599609375;-0.3984105650857865388303480358445085585117340087890625;0.0248539662468534316985824261792004108428955078125;-0.5565515333466073411017305261339060962200164794921875;-0.95889856787881289079678026610054075717926025390625;-0.4240370649953770776363626282545737922191619873046875;-0.154762613758491429649666315526701509952545166015625;-0.5293972412672884875206591459573246538639068603515625;-0.8218871603139756842892893473617732524871826171875;0.902172162739297345268596473033539950847625732421875;0.1644243969484582290618845945573411881923675537109375;-0.25660351976978379440197386429645121097564697265625]
      mask Display: e = 0.06;c1 = [120 150 230]/255;c2 = ([120 150 230]+0)/383;c3 = ([120 150 230]+128)/383;patch([0 1 1 0],[0 0 1 1],c1);patch([0 1 1 1-e 1-e 0+e],[0 0 1 1-e 0+e 0+e],c2);patch([0 0 1 1-e 0+e 0+e],[0 1 1 1-e 1-e 0+e],c3);plot([0 1 1 0 0],[0 0 1 1 0]);disp('weights');
  "IW{2,1}(6,:)'" : Constant  Value=[0.763625787908121633762448254856280982494354248046875;-0.510238191894798465142457644105888903141021728515625;0.0539282061626591424641219418845139443874359130859375;-0.1081407596574124330146560168941505253314971923828125;-0.698406224015539311977818215382285416126251220703125;0.885866835405014096949116719770245254039764404296875;0.30471455909570810405284646549262106418609619140625;-0.1742765867999820361688989578397013247013092041015625;0.79895722311737582543855751282535493373870849609375;-0.500258731271066015011683703050948679447174072265625;0.5833950698598420192553248853073455393314361572265625;-0.0050891584928611788285479633486829698085784912109375;0.8483095897888885961179994410485960543155670166015625;-0.95031539270193920998508474440313875675201416015625;-0.88749389934290690007401281036436557769775390625;-0.9916936303423813381385798493283800780773162841796875;-0.206946505607646713542635552585124969482421875;-0.2686219046287907641357151078409515321254730224609375;-0.203162032604441211702805958339013159275054931640625;-0.0969272154339890779084498717566020786762237548828125]
      mask Display: e = 0.06;c1 = [120 150 230]/255;c2 = ([120 150 230]+0)/383;c3 = ([120 150 230]+128)/383;patch([0 1 1 0],[0 0 1 1],c1);patch([0 1 1 1-e 1-e 0+e],[0 0 1 1-e 0+e 0+e],c2);patch([0 0 1 1-e 0+e 0+e],[0 1 1 1-e 1-e 0+e],c3);plot([0 1 1 0 0],[0 0 1 1 0]);disp('weights');
  "IW{2,1}(7,:)'" : Constant  Value=[0.243816580319846265556549269604147411882877349853515625;0.06340244036734686561285201378268538974225521087646484375;0.9893117684012364687617946401587687432765960693359375;-0.005559528978159367085254416451789438724517822265625;0.358795542961496349843031339332810603082180023193359375;0.31317562167653523186316988358157686889171600341796875;-0.935978356470393624277903654729016125202178955078125;-0.62532194046897926487105223714024759829044342041015625;-0.464494065599977634661854608566500246524810791015625;-0.2522222217247429565389893468818627297878265380859375;0.9839425478357648469085461329086683690547943115234375;-0.81466316780665781749348752782680094242095947265625;-0.37961746810823926434608210911392234265804290771484375;-0.8848200603310136802548413470503874123096466064453125;0.4598860045009038888252916876808740198612213134765625;0.603482924821817423577385852695442736148834228515625;-0.668634886838280095844311290420591831207275390625;0.100201642029997817218145428341813385486602783203125;-0.443393888126671964489133870301884599030017852783203125;-0.393579329364300456450820320242200978100299835205078125]
      mask Display: e = 0.06;c1 = [120 150 230]/255;c2 = ([120 150 230]+0)/383;c3 = ([120 150 230]+128)/383;patch([0 1 1 0],[0 0 1 1],c1);patch([0 1 1 1-e 1-e 0+e],[0 0 1 1-e 0+e 0+e],c2);patch([0 0 1 1-e 0+e 0+e],[0 1 1 1-e 1-e 0+e],c3);plot([0 1 1 0 0],[0 0 1 1 0]);disp('weights');
  "IW{2,1}(8,:)'" : Constant  Value=[0.3573704202167637955511736436164937913417816162109375;-0.16638718242525840640411161075462587177753448486328125;0.482027928235543523527439901954494416713714599609375;0.482486092005906030966144726335187442600727081298828125;0.52951517334978370765696809030487202107906341552734375;-0.84171464494981318438249218161217868328094482421875;0.1293726842827168932448245186606072820723056793212890625;-0.8372370805084179412602907177642919123172760009765625;-0.3259895821479528166264572064392268657684326171875;0.240830678318555424510805096360854804515838623046875;-0.4242556894882978379968108129105530679225921630859375;0.1324277373689088932451340951956808567047119140625;0.41353997604249725927871850217343308031558990478515625;0.146813592451838115238160753506235778331756591796875;-0.5029809805158951263592825853265821933746337890625;0.6494222698706695329207150280126370489597320556640625;-0.49521646019381704295625468148500658571720123291015625;-0.48398271571584405847943344269879162311553955078125;0.498458004296726542303730411731521598994731903076171875;-0.99977096742259241590744522909517399966716766357421875]
      mask Display: e = 0.06;c1 = [120 150 230]/255;c2 = ([120 150 230]+0)/383;c3 = ([120 150 230]+128)/383;patch([0 1 1 0],[0 0 1 1],c1);patch([0 1 1 1-e 1-e 0+e],[0 0 1 1-e 0+e 0+e],c2);patch([0 0 1 1-e 0+e 0+e],[0 1 1 1-e 1-e 0+e],c3);plot([0 1 1 0 0],[0 0 1 1 0]);disp('weights');
  "IW{2,1}(9,:)'" : Constant  Value=[-0.29994247694269293713631441278266720473766326904296875;0.94175125883584021035943578681326471269130706787109375;0.62791242131358959710496492334641516208648681640625;0.416965076456069561050554739267681725323200225830078125;0.6440231750254070686168006432126276195049285888671875;-0.171954839111356727610058214850141666829586029052734375;-0.8920475073956921630013994217733852565288543701171875;-0.44426145419573936923285373268299736082553863525390625;-0.6812133662366768316331899768556468188762664794921875;0.55170432766943466873499346547760069370269775390625;0.80806581745568717423111593234352767467498779296875;0.6887267075925855852602808226947672665119171142578125;-0.32920325044988596463468866204493679106235504150390625;0.8556078203530879111582407858804799616336822509765625;-0.69499866597627069086939854969386942684650421142578125;-0.2268043242924691060835584721644409000873565673828125;-0.25451256596413684984980818626354448497295379638671875;0.2110391620766784992468956261291168630123138427734375;-0.32071433627852885539510907619842328131198883056640625;-0.55016587764656177395039549082866869866847991943359375]
      mask Display: e = 0.06;c1 = [120 150 230]/255;c2 = ([120 150 230]+0)/383;c3 = ([120 150 230]+128)/383;patch([0 1 1 0],[0 0 1 1],c1);patch([0 1 1 1-e 1-e 0+e],[0 0 1 1-e 0+e 0+e],c2);patch([0 0 1 1-e 0+e 0+e],[0 1 1 1-e 1-e 0+e],c3);plot([0 1 1 0 0],[0 0 1 1 0]);disp('weights');
  Mux : Mux  Inputs=20
      mask Display: e = 0.06;c1 = [120 150 230]/255;c2 = ([120 150 230]+0)/383;c3 = ([120 150 230]+128)/383;patch([0 1 1 0],[0 0 1 1],c1);patch([0 1 1 1-e 1-e 0+e],[0 0 1 1-e 0+e 0+e],c2);patch([0 0 1 1-e 0+e 0+e],[0 1 1 1-e 1-e 0+e],c3);plot([0 1 1 0 0],[0 0 1 1 0]);disp('Mux');
  dotprod{1..20} (20 alike) : neural/Weight Functions/dotprod
  "lz{2,1}" : Outport
      mask Display: e = 0.06;c1 = [120 230 180]/255;c2 = ([120 230 180]+0)/(256+128);c3 = ([120 230 180]+128)/(256+128);patch([0 1 1 0],[0 0 1 1],c1);patch([0 1 1 1-e 1-e 0+e],[0 0 1 1-e 0+e 0+e],c2);patch([0 0 1 1-e 0+e 0+e],[0 1 1 1-e 1-e 0+e],c3);plot([0 1 1 0 0],[0 0 1 1 0]);
  wires:
  "IW{2,1}(1,:)'"/1 -> dotprod1/1
  "ad{2,1}"/1 -> dotprod1/2, dotprod2/2, dotprod3/2, dotprod4/2, dotprod5/2, dotprod6/2, dotprod7/2, dotprod8/2, dotprod9/2, dotprod10/2, dotprod11/2, dotprod12/2, dotprod13/2, dotprod14/2, dotprod15/2, dotprod16/2, dotprod17/2, dotprod18/2, dotprod19/2, dotprod20/2
  dotprod1/1 -> Mux/1
  "IW{2,1}(2,:)'"/1 -> dotprod2/1
  dotprod2/1 -> Mux/2
  "IW{2,1}(3,:)'"/1 -> dotprod3/1
  dotprod3/1 -> Mux/3
  "IW{2,1}(4,:)'"/1 -> dotprod4/1
  dotprod4/1 -> Mux/4
  "IW{2,1}(5,:)'"/1 -> dotprod5/1
  dotprod5/1 -> Mux/5
  "IW{2,1}(6,:)'"/1 -> dotprod6/1
  dotprod6/1 -> Mux/6
  "IW{2,1}(7,:)'"/1 -> dotprod7/1
  dotprod7/1 -> Mux/7
  "IW{2,1}(8,:)'"/1 -> dotprod8/1
  dotprod8/1 -> Mux/8
  "IW{2,1}(9,:)'"/1 -> dotprod9/1
  dotprod9/1 -> Mux/9
  "IW{2,1}(10,:)'"/1 -> dotprod10/1
  dotprod10/1 -> Mux/10
  "IW{2,1}(11,:)'"/1 -> dotprod11/1
  dotprod11/1 -> Mux/11
  "IW{2,1}(12,:)'"/1 -> dotprod12/1
  dotprod12/1 -> Mux/12
  "IW{2,1}(13,:)'"/1 -> dotprod13/1
  dotprod13/1 -> Mux/13
  "IW{2,1}(14,:)'"/1 -> dotprod14/1
  dotprod14/1 -> Mux/14
  "IW{2,1}(15,:)'"/1 -> dotprod15/1
  dotprod15/1 -> Mux/15
  "IW{2,1}(16,:)'"/1 -> dotprod16/1
  dotprod16/1 -> Mux/16
  "IW{2,1}(17,:)'"/1 -> dotprod17/1
  dotprod17/1 -> Mux/17
  "IW{2,1}(18,:)'"/1 -> dotprod18/1
  dotprod18/1 -> Mux/18
  "IW{2,1}(19,:)'"/1 -> dotprod19/1
  dotprod19/1 -> Mux/19
  "IW{2,1}(20,:)'"/1 -> dotprod20/1
  dotprod20/1 -> Mux/20
  Mux/1 -> "lz{2,1}"/1

== system nn_fuel_control_4_20/Air Fuel Control Model 1/Feed-Forward Neural Network/Layer 3/Delays 1 ==
  "p{3}" : Inport  PortDimensions=20
      mask Display: e = 0.06;c1 = [120 230 180]/255;c2 = ([120 230 180]+0)/(256+128);c3 = ([120 230 180]+128)/(256+128);patch([0 1 1 0],[0 0 1 1],c1);patch([0 1 1 1-e 1-e 0+e],[0 0 1 1-e 0+e 0+e],c2);patch([0 0 1 1-e 0+e 0+e],[0 1 1 1-e 1-e 0+e],c3);plot([0 1 1 0 0],[0 0 1 1 0]);
  mux : Mux  Inputs=1
      mask Display: e = 0.06;c1 = [120 150 230]/255;c2 = ([120 150 230]+0)/383;c3 = ([120 150 230]+128)/383;patch([0 1 1 0],[0 0 1 1],c1);patch([0 1 1 1-e 1-e 0+e],[0 0 1 1-e 0+e 0+e],c2);patch([0 0 1 1-e 0+e 0+e],[0 1 1 1-e 1-e 0+e],c3);plot([0 1 1 0 0],[0 0 1 1 0]);disp('Mux')
  "pd{3,2}" : Outport
      mask Display: e = 0.06;c1 = [120 230 180]/255;c2 = ([120 230 180]+0)/(256+128);c3 = ([120 230 180]+128)/(256+128);patch([0 1 1 0],[0 0 1 1],c1);patch([0 1 1 1-e 1-e 0+e],[0 0 1 1-e 0+e 0+e],c2);patch([0 0 1 1-e 0+e 0+e],[0 1 1 1-e 1-e 0+e],c3);plot([0 1 1 0 0],[0 0 1 1 0]);
  wires:
  "p{3}"/1 -> mux/1
  mux/1 -> "pd{3,2}"/1
